simulink model "gm_CustArch_v13"  (R2020a)
settings: Solver=FixedStepDiscrete  StartTime=0.0  StopTime=840000  RelTol=1e-3
libraries: simulink x89, hdlsllib x54, hdlmdlgenlib x25
(part 2 of 3)

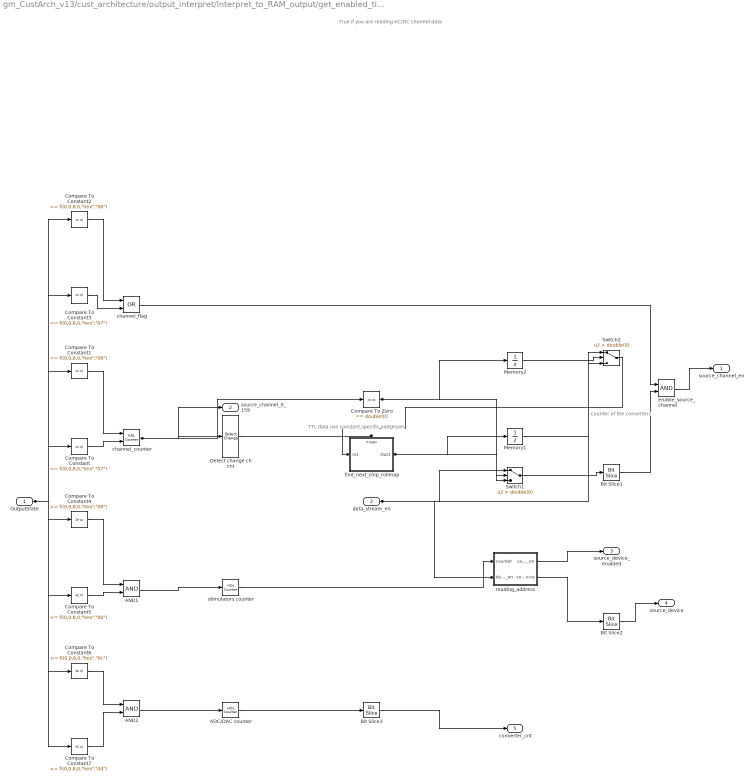
== system gm_CustArch_v13/cust_architecture/output_interpret/Interpret_to_RAM_output/get_enabled_timings  ==
  note: counter of the converters
  note: TTL data use constant specific addresses
  note: True if you are reading AC/DC channel data
  OutputState : Inport  OutDataTypeStr=uint8  PortDimensions=1  SampleTime=1
  data_stream_en : Inport  Port=2  OutDataTypeStr=uint8  PortDimensions=1  SampleTime=1
  ADC/DAC counter : hdlsllib/Sources/HDL Counter  CountType=Count limited  CountInit=double(0)  CountStep=double(1)  CountMax=double(7)  CountFromType=Initial value  CountFrom=double(0)  CountResetPort=off  CountLoadPort=off  CountEnbPort=on  CountDirPort=off  CountDataType=Unsigned  CountWordLen=8  CountFracLen=0  CountSampTime=1
  AND1 : Logic  AllPortsSameDT=off  OutDataTypeStr=boolean  SampleTime=1
  AND2 : Logic  AllPortsSameDT=off  OutDataTypeStr=boolean  SampleTime=1
  Bit Slice1 : hdlsllib/Logic and Bit Operations/Bit Slice  lidx=double(0)  ridx=double(0)
      settings: SourceProductBaseCode=SL
  Bit Slice2 : hdlsllib/Logic and Bit Operations/Bit Slice  lidx=double(2)  ridx=double(0)
      settings: SourceProductBaseCode=SL
  Bit Slice3 : hdlsllib/Logic and Bit Operations/Bit Slice  lidx=double(2)  ridx=double(0)
      settings: SourceProductBaseCode=SL
  Compare To Constant : simulink/Logic and Bit Operations/Compare To Constant  relop===  const="fi(0,0,8,0,\"hex\",\"07\")"  OutDataTypeStr=boolean
  Compare To Constant1 : simulink/Logic and Bit Operations/Compare To Constant  relop===  const="fi(0,0,8,0,\"hex\",\"08\")"  OutDataTypeStr=boolean
  Compare To Constant2 : simulink/Logic and Bit Operations/Compare To Constant  relop===  const="fi(0,0,8,0,\"hex\",\"06\")"  OutDataTypeStr=boolean
  Compare To Constant3 : simulink/Logic and Bit Operations/Compare To Constant  relop===  const="fi(0,0,8,0,\"hex\",\"07\")"  OutDataTypeStr=boolean
  Compare To Constant4 : simulink/Logic and Bit Operations/Compare To Constant  relop=>=  const="fi(0,0,8,0,\"hex\",\"08\")"  OutDataTypeStr=boolean
  Compare To Constant5 : simulink/Logic and Bit Operations/Compare To Constant  relop=<=  const="fi(0,0,8,0,\"hex\",\"0b\")"  OutDataTypeStr=boolean
  Compare To Constant6 : simulink/Logic and Bit Operations/Compare To Constant  relop=>=  const="fi(0,0,8,0,\"hex\",\"0c\")"  OutDataTypeStr=boolean
  Compare To Constant7 : simulink/Logic and Bit Operations/Compare To Constant  relop=<=  const="fi(0,0,8,0,\"hex\",\"0d\")"  OutDataTypeStr=boolean
  Compare To Zero : simulink/Logic and Bit Operations/Compare To Constant  relop===  const=double(0)  OutDataTypeStr=boolean
  Detect change ch cnt : simulink/Logic and Bit Operations/Detect Change  vinit=0  OutDataTypeStr=boolean
  Memory1 : UnitDelay  InitialCondition=double(0)  SampleTime=1
  Memory2 : UnitDelay  InitialCondition=double(0)  SampleTime=1
  Switch1 : Switch  Criteria=u2 > Threshold  Threshold=double(0)  OutDataTypeStr=uint8  SampleTime=1
  Switch2 : Switch  Criteria=u2 > Threshold  Threshold=double(0)  OutDataTypeStr=uint8  SampleTime=1
  channel_counter : hdlsllib/Sources/HDL Counter  CountType=Count limited  CountInit=double(0)  CountStep=double(1)  CountMax=double(159)  CountFromType=Initial value  CountFrom=double(0)  CountResetPort=on  CountLoadPort=off  CountEnbPort=on  CountDirPort=off  CountDataType=Unsigned  CountWordLen=8  CountFracLen=0  CountSampTime=1
  channel_flag : Logic  Operator=OR  AllPortsSameDT=off  OutDataTypeStr=boolean  SampleTime=1
  enable_source_channel : Logic  AllPortsSameDT=off  OutDataTypeStr=boolean  SampleTime=1
  find_next_chip_rollmap : Subsystem
  reading_address : Subsystem
  stimulators counter : hdlsllib/Sources/HDL Counter  CountType=Count limited  CountInit=double(0)  CountStep=double(1)  CountMax=double(7)  CountFromType=Initial value  CountFrom=double(0)  CountResetPort=off  CountLoadPort=off  CountEnbPort=on  CountDirPort=off  CountDataType=Unsigned  CountWordLen=8  CountFracLen=0  CountSampTime=1
  source_channel_en : Outport  VectorParamsAs1DForOutWhenUnconnected=off
  source_channel_0_159 : Outport  Port=2  OutMin=0  OutMax=159  OutDataTypeStr=uint8  VectorParamsAs1DForOutWhenUnconnected=off  LockScale=on
  source_device_enabled : Outport  Port=3  VectorParamsAs1DForOutWhenUnconnected=off
  source_device : Outport  Port=4  VectorParamsAs1DForOutWhenUnconnected=off
  converter_cnt : Outport  Port=5  VectorParamsAs1DForOutWhenUnconnected=off
  wires:
  OutputState/1 -> Compare To Constant7/1, Compare To Constant6/1, Compare To Constant5/1, Compare To Constant4/1, Compare To Constant3/1, Compare To Constant2/1, Compare To Constant1/1, Compare To Constant/1
  data_stream_en/1 -> Switch2/1, Switch1/1, reading_address/2(data_stream_en)
  ADC/DAC counter/1 -> Bit Slice3/1
  AND1/1 -> stimulators counter/1
  AND2/1 -> ADC/DAC counter/1
  Bit Slice1/1 -> enable_source_channel/2
  Bit Slice2/1 -> source_device/1
  Bit Slice3/1 -> converter_cnt/1
  Compare To Constant/1 -> channel_counter/2
  Compare To Constant1/1 -> channel_counter/1
  Compare To Constant2/1 -> channel_flag/1
  Compare To Constant3/1 -> channel_flag/2
  Compare To Constant4/1 -> AND1/1
  Compare To Constant5/1 -> AND1/2
  Compare To Constant6/1 -> AND2/1
  Compare To Constant7/1 -> AND2/2
  Compare To Zero/1 -> Switch1/2, Memory2/1
  Detect change ch cnt/1 -> find_next_chip_rollmap/Trigger
  Memory1/1 -> Switch2/3
  Memory2/1 -> Switch2/2
  Switch1/1 -> Bit Slice1/1
  Switch2/1 -> find_next_chip_rollmap/1(In1)
  channel_counter/1 -> Compare To Zero/1, Detect change ch cnt/1, source_channel_0_159/1
  channel_flag/1 -> enable_source_channel/1
  enable_source_channel/1 -> source_channel_en/1
  find_next_chip_rollmap/1(Out1) -> Switch1/3, Memory1/1
  reading_address/1(source_device_en) -> source_device_enabled/1
  reading_address/2(source_device) -> Bit Slice2/1
  stimulators counter/1 -> reading_address/1("counter ")

== system gm_CustArch_v13/cust_architecture/process_and_retrieve/Filter_ch1/digital_filter ==
  raw_input : Inport  OutDataTypeStr=uint16  PortDimensions=[8 1]  SampleTime=1  LockScale=on
  Enable : Inport  Port=2  OutDataTypeStr=boolean  SampleTime=1
  Add : Sum  Inputs=+-  AccumDataTypeStr=fixdt(1, 17, 0)  OutDataTypeStr=fixdt(1, 32, 16)  SampleTime=1
  Add1 : Sum  AccumDataTypeStr=fixdt(1, 38, 20)  OutDataTypeStr=uint16  SampleTime=1
  Add1_out1bypassMux : MultiPortSwitch  DataPortOrder=Zero-based contiguous  Inputs=2  zeroidx=on  OutDataTypeStr=uint16  SampleTime=1
  Constant : Constant  Value=32768  OutDataTypeStr=uint16  SampleTime=1
  Constant1 : Constant  Value=32768  OutDataTypeStr=uint16  SampleTime=1
  filter_output_bypass : UnitDelay  SampleTime=1
  highpass : Subsystem
  filter_output : Outport  InitialOutput=0  LockScale=on
  wires:
  Enable/1 -> Add1_out1bypassMux/1, highpass/2(Enable_out2)
  raw_input/1 -> Add/1
  Add/1 -> highpass/1(In)
  Add1/1 -> Add1_out1bypassMux/3
  Constant/1 -> Add/2
  Constant1/1 -> Add1/2
  highpass/1(Out) -> Add1/1
  Add1_out1bypassMux/1 -> filter_output_bypass/1, filter_output/1
  filter_output_bypass/1 -> Add1_out1bypassMux/2

== system gm_CustArch_v13/cust_architecture/input_interpret_store_retrieve/Interpret_to_RAM_input/interpret incoming data/condition to count DAC or ADC  ==
  fifo_write_to : Inport  OutDataTypeStr=boolean  PortDimensions=1  SampleTime=1
  input_state : Inport  Port=2  OutDataTypeStr=uint8  PortDimensions=1  SampleTime=1
  AND : Logic  AllPortsSameDT=off  OutDataTypeStr=boolean  SampleTime=1
  OR : Logic  Operator=OR  AllPortsSameDT=off  OutDataTypeStr=boolean  SampleTime=1
  is state_ADC : simulink/Logic and Bit Operations/Compare To Constant  relop===  const="fi(0,0,8,0,\"hex\",\"0d\")"  OutDataTypeStr=boolean
  is state_DAC : simulink/Logic and Bit Operations/Compare To Constant  relop===  const="fi(0,0,8,0,\"hex\",\"0c\")"  OutDataTypeStr=boolean
  Out1 : Outport  VectorParamsAs1DForOutWhenUnconnected=off
  wires:
  fifo_write_to/1 -> AND/1
  input_state/1 -> is state_DAC/1, is state_ADC/1
  AND/1 -> Out1/1
  OR/1 -> AND/2
  is state_ADC/1 -> OR/2
  is state_DAC/1 -> OR/1

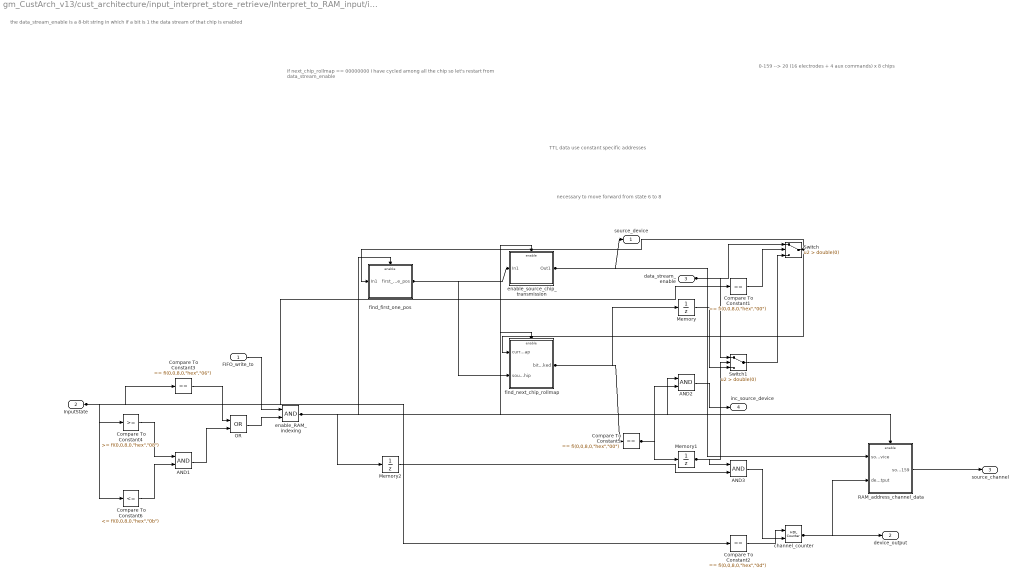
== system gm_CustArch_v13/cust_architecture/input_interpret_store_retrieve/Interpret_to_RAM_input/interpret incoming data/get_sources_and_RAM_addresses ==
  note: TTL data use constant specific addresses
  note: the data_stream_enable is a 8-bit string in which if a bit is 1 the data stream of that chip is enabled
  note: if next_chip_rollmap == 00000000 I have cycled among all the chip so let's restart from data_stream_enable
  note: 0-159 --> 20 (16 electrodes + 4 aux commands) x 8 chips
  note: necessary to move forward from state 6 to 8
  FIFO_write_to : Inport  OutDataTypeStr=boolean  PortDimensions=1  SampleTime=1
  InputState : Inport  Port=2  OutDataTypeStr=uint8  PortDimensions=1  SampleTime=1
  data_stream_enable : Inport  Port=3  OutDataTypeStr=uint8  PortDimensions=1  SampleTime=1
  AND1 : Logic  AllPortsSameDT=off  OutDataTypeStr=boolean  SampleTime=1
  AND2 : Logic  AllPortsSameDT=off  OutDataTypeStr=boolean  SampleTime=1
  AND3 : Logic  AllPortsSameDT=off  OutDataTypeStr=boolean  SampleTime=1
  Compare To Constant1 : simulink/Logic and Bit Operations/Compare To Constant  relop===  const="fi(0,0,8,0,\"hex\",\"00\")"  OutDataTypeStr=boolean
  Compare To Constant2 : simulink/Logic and Bit Operations/Compare To Constant  relop===  const="fi(0,0,8,0,\"hex\",\"0d\")"  OutDataTypeStr=boolean
  Compare To Constant3 : simulink/Logic and Bit Operations/Compare To Constant  relop===  const="fi(0,0,8,0,\"hex\",\"06\")"  OutDataTypeStr=boolean
  Compare To Constant4 : simulink/Logic and Bit Operations/Compare To Constant  relop=>=  const="fi(0,0,8,0,\"hex\",\"08\")"  OutDataTypeStr=boolean
  Compare To Constant5 : simulink/Logic and Bit Operations/Compare To Constant  relop===  const="fi(0,0,8,0,\"hex\",\"00\")"  OutDataTypeStr=boolean
  Compare To Constant6 : simulink/Logic and Bit Operations/Compare To Constant  relop=<=  const="fi(0,0,8,0,\"hex\",\"0b\")"  OutDataTypeStr=boolean
  Memory : UnitDelay  InitialCondition=double(0)  SampleTime=1
  Memory1 : UnitDelay  InitialCondition=double(0)  SampleTime=1
  Memory2 : UnitDelay  InitialCondition=double(0)  SampleTime=1
  OR : Logic  Operator=OR  AllPortsSameDT=off  OutDataTypeStr=boolean  SampleTime=1
  RAM_address_channel_data : Subsystem
  Switch : Switch  Criteria=u2 > Threshold  Threshold=double(0)  OutDataTypeStr=uint8  SampleTime=1
  Switch1 : Switch  Criteria=u2 > Threshold  Threshold=double(0)  OutDataTypeStr=uint8  SampleTime=1
  channel_counter : hdlsllib/Sources/HDL Counter  CountType=Count limited  CountInit=double(0)  CountStep=double(1)  CountMax=double(20)  CountFromType=Initial value  CountFrom=double(0)  CountResetPort=on  CountLoadPort=off  CountEnbPort=on  CountDirPort=off  CountDataType=Unsigned  CountWordLen=8  CountFracLen=0  CountSampTime=1
  enable_RAM_indexing : Logic  AllPortsSameDT=off  OutDataTypeStr=boolean  SampleTime=1
  enable_source_chip_transmission : Subsystem
  find_first_one_pos : Subsystem
  find_next_chip_rollmap : Subsystem
  source_device : Outport  VectorParamsAs1DForOutWhenUnconnected=off
  device_output : Outport  Port=2  VectorParamsAs1DForOutWhenUnconnected=off
  source_channel : Outport  Port=3  VectorParamsAs1DForOutWhenUnconnected=off
  inc_source_device : Outport  Port=4  VectorParamsAs1DForOutWhenUnconnected=off
  wires:
  FIFO_write_to/1 -> enable_RAM_indexing/1
  InputState/1 -> Compare To Constant6/1, Compare To Constant4/1, Compare To Constant3/1, Compare To Constant2/1, Compare To Constant1/1
  data_stream_enable/1 -> Switch1/1, Switch/1
  AND1/1 -> OR/2
  AND2/1 -> inc_source_device/1
  AND3/1 -> channel_counter/2
  Compare To Constant1/1 -> Switch/2
  Compare To Constant2/1 -> channel_counter/1
  Compare To Constant3/1 -> OR/1
  Compare To Constant4/1 -> AND1/1
  Compare To Constant5/1 -> AND2/2, Memory1/1
  Compare To Constant6/1 -> AND1/2
  Memory/1 -> Switch1/3
  Memory1/1 -> Switch1/2, AND3/1
  Memory2/1 -> AND3/2
  OR/1 -> enable_RAM_indexing/2
  RAM_address_channel_data/1(source_channel_0_159) -> source_channel/1
  Switch/1 -> find_next_chip_rollmap/1(curr_chip_rollmap), find_first_one_pos/1(In1)
  Switch1/1 -> Switch/3
  channel_counter/1 -> device_output/1, RAM_address_channel_data/2(dev_output)
  enable_RAM_indexing/1 -> AND2/1, Memory2/1, enable_source_chip_transmission/Enable, RAM_address_channel_data/Enable, find_next_chip_rollmap/Enable, find_first_one_pos/Enable
  enable_source_chip_transmission/1(Out1) -> source_device/1, RAM_address_channel_data/1(source_device)
  find_first_one_pos/1(first_one_pos) -> enable_source_chip_transmission/1(In1), find_next_chip_rollmap/2(source_chip)
  find_next_chip_rollmap/1(bit_masked) -> Compare To Constant5/1, Memory/1

== system gm_CustArch_v13/cust_architecture/output_interpret/Interpret_to_RAM_output/get_enabled_timings /find_next_chip_rollmap ==
  In1 : Inport  OutDataTypeStr=uint8  PortDimensions=1
  Trigger : TriggerPort  VariantControl=(inherit)  PortDimensions=1  OutDataTypeStr=boolean
  Bit Rotate : hdlsllib/Logic and Bit Operations/Bit Rotate  mode=Rotate Right  N=double(1)
      settings: SourceProductBaseCode=SL
  Out1 : Outport  InitialOutput=0  VectorParamsAs1DForOutWhenUnconnected=off
  wires:
  In1/1 -> Bit Rotate/1
  Bit Rotate/1 -> Out1/1

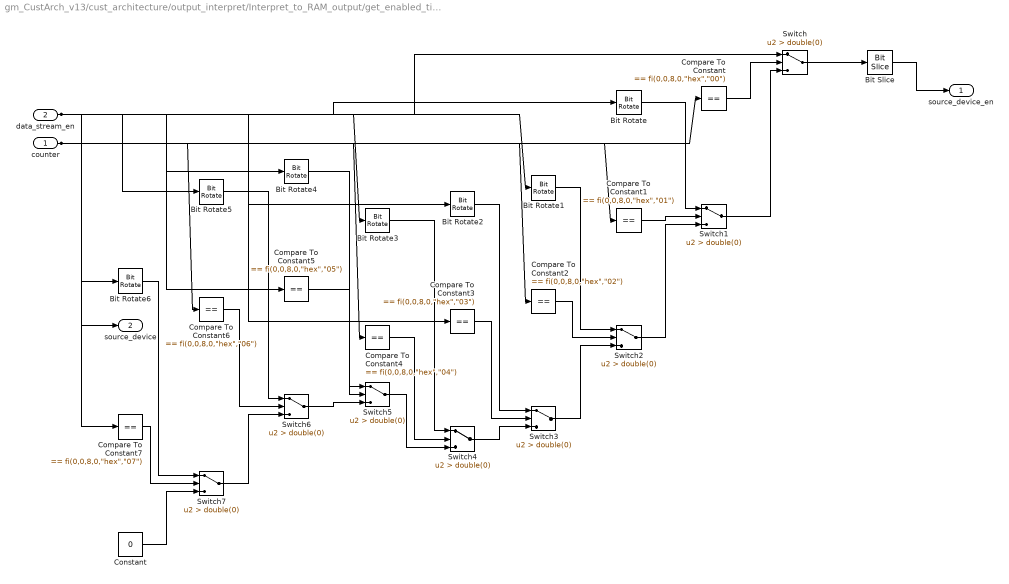
== system gm_CustArch_v13/cust_architecture/output_interpret/Interpret_to_RAM_output/get_enabled_timings /reading_address ==
  "counter " : Inport  OutDataTypeStr=uint8  PortDimensions=1  SampleTime=1
  data_stream_en : Inport  Port=2  OutDataTypeStr=uint8  PortDimensions=1  SampleTime=1
  Bit Rotate : hdlsllib/Logic and Bit Operations/Bit Rotate  mode=Rotate Right  N=double(1)
      settings: SourceProductBaseCode=SL
  Bit Rotate1 : hdlsllib/Logic and Bit Operations/Bit Rotate  mode=Rotate Right  N=double(2)
      settings: SourceProductBaseCode=SL
  Bit Rotate2 : hdlsllib/Logic and Bit Operations/Bit Rotate  mode=Rotate Right  N=double(3)
      settings: SourceProductBaseCode=SL
  Bit Rotate3 : hdlsllib/Logic and Bit Operations/Bit Rotate  mode=Rotate Right  N=double(4)
      settings: SourceProductBaseCode=SL
  Bit Rotate4 : hdlsllib/Logic and Bit Operations/Bit Rotate  mode=Rotate Right  N=double(5)
      settings: SourceProductBaseCode=SL
  Bit Rotate5 : hdlsllib/Logic and Bit Operations/Bit Rotate  mode=Rotate Right  N=double(6)
      settings: SourceProductBaseCode=SL
  Bit Rotate6 : hdlsllib/Logic and Bit Operations/Bit Rotate  mode=Rotate Right  N=double(7)
      settings: SourceProductBaseCode=SL
  Bit Slice : hdlsllib/Logic and Bit Operations/Bit Slice  lidx=double(0)  ridx=double(0)
      settings: SourceProductBaseCode=SL
  Compare To Constant : simulink/Logic and Bit Operations/Compare To Constant  relop===  const="fi(0,0,8,0,\"hex\",\"00\")"  OutDataTypeStr=boolean
  Compare To Constant1 : simulink/Logic and Bit Operations/Compare To Constant  relop===  const="fi(0,0,8,0,\"hex\",\"01\")"  OutDataTypeStr=boolean
  Compare To Constant2 : simulink/Logic and Bit Operations/Compare To Constant  relop===  const="fi(0,0,8,0,\"hex\",\"02\")"  OutDataTypeStr=boolean
  Compare To Constant3 : simulink/Logic and Bit Operations/Compare To Constant  relop===  const="fi(0,0,8,0,\"hex\",\"03\")"  OutDataTypeStr=boolean
  Compare To Constant4 : simulink/Logic and Bit Operations/Compare To Constant  relop===  const="fi(0,0,8,0,\"hex\",\"04\")"  OutDataTypeStr=boolean
  Compare To Constant5 : simulink/Logic and Bit Operations/Compare To Constant  relop===  const="fi(0,0,8,0,\"hex\",\"05\")"  OutDataTypeStr=boolean
  Compare To Constant6 : simulink/Logic and Bit Operations/Compare To Constant  relop===  const="fi(0,0,8,0,\"hex\",\"06\")"  OutDataTypeStr=boolean
  Compare To Constant7 : simulink/Logic and Bit Operations/Compare To Constant  relop===  const="fi(0,0,8,0,\"hex\",\"07\")"  OutDataTypeStr=boolean
  Constant : Constant  Value=0  OutDataTypeStr=uint8  SampleTime=1
  Switch{,1..7} (8 alike) : Switch  Criteria=u2 > Threshold  Threshold=double(0)  OutDataTypeStr=uint8  SampleTime=1
  source_device_en : Outport  VectorParamsAs1DForOutWhenUnconnected=off
  source_device : Outport  Port=2  VectorParamsAs1DForOutWhenUnconnected=off
  wires:
  "counter "/1 -> Compare To Constant7/1, Compare To Constant6/1, Compare To Constant5/1, Compare To Constant4/1, Compare To Constant3/1, Compare To Constant2/1, Compare To Constant1/1, Compare To Constant/1, source_device/1
  data_stream_en/1 -> Switch/1, Bit Rotate6/1, Bit Rotate5/1, Bit Rotate4/1, Bit Rotate3/1, Bit Rotate2/1, Bit Rotate1/1, Bit Rotate/1
  Bit Rotate/1 -> Switch1/1
  Bit Rotate1/1 -> Switch2/1
  Bit Rotate2/1 -> Switch3/1
  Bit Rotate3/1 -> Switch4/1
  Bit Rotate4/1 -> Switch5/1
  Bit Rotate5/1 -> Switch6/1
  Bit Rotate6/1 -> Switch7/1
  Bit Slice/1 -> source_device_en/1
  Compare To Constant/1 -> Switch/2
  Compare To Constant1/1 -> Switch1/2
  Compare To Constant2/1 -> Switch2/2
  Compare To Constant3/1 -> Switch3/2
  Compare To Constant4/1 -> Switch4/2
  Compare To Constant5/1 -> Switch5/2
  Compare To Constant6/1 -> Switch6/2
  Compare To Constant7/1 -> Switch7/2
  Constant/1 -> Switch7/3
  Switch/1 -> Bit Slice/1
  Switch1/1 -> Switch/3
  Switch2/1 -> Switch1/3
  Switch3/1 -> Switch2/3
  Switch4/1 -> Switch3/3
  Switch5/1 -> Switch4/3
  Switch6/1 -> Switch5/3
  Switch7/1 -> Switch6/3

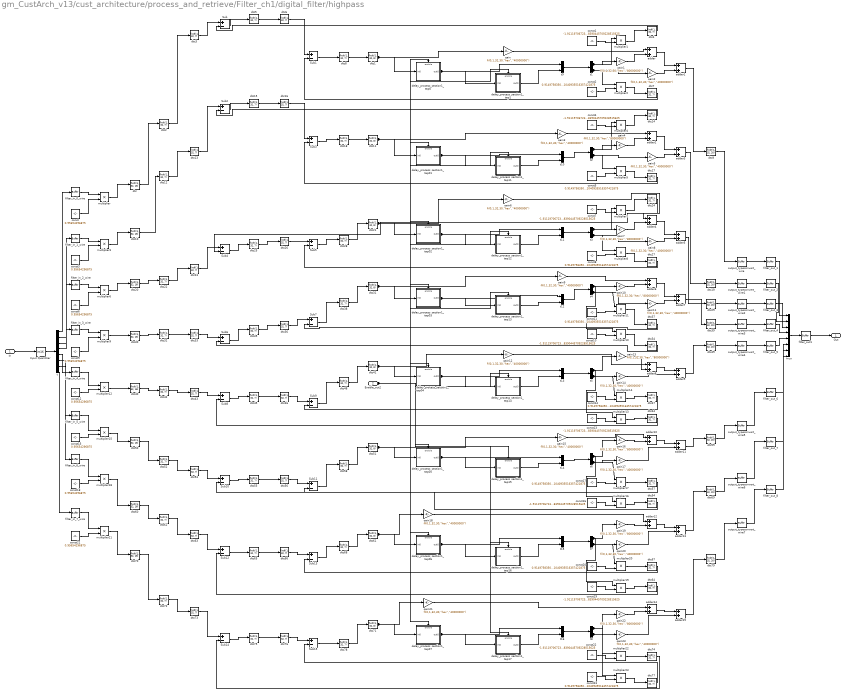
== system gm_CustArch_v13/cust_architecture/process_and_retrieve/Filter_ch1/digital_filter/highpass ==
  In : Inport  OutDataTypeStr=fixdt(1, 32, 16)  PortDimensions=[8 1]  SampleTime=1
  Enable_out2 : Inport  Port=2  OutDataTypeStr=boolean  SampleTime=1
  Input Quantizer : DataTypeConversion  OutDataTypeStr=int16  RndMeth=Round  SampleTime=1  SaturateOnIntegerOverflow=on
  Sub{,1..15} (16 alike) : Sum  Inputs=+-  OutDataTypeStr=fixdt(1, 33, 7)  RndMeth=Nearest  SaturateOnIntegerOverflow=on  SampleTime=1
  adder{,1..15} (16 alike) : Sum  OutDataTypeStr=fixdt(1, 32, 7)  RndMeth=Nearest  SaturateOnIntegerOverflow=on  SampleTime=1
  const{,3,6,9,12,15,18,21} (8 alike) : Constant  Value=0.95654296875  OutDataTypeStr=fixdt(1, 32, 15)  SampleTime=1
  const{1,4,7,10,13,16,19,22} (8 alike) : Constant  Value=-1.911197067238390445709228515625  OutDataTypeStr=fixdt(1, 32, 30)  SampleTime=1
  const{2,5,8,11,14,17,20,23} (8 alike) : Constant  Value=0.91497583501040935516357421875  OutDataTypeStr=fixdt(1, 32, 30)  SampleTime=1
  delay_process_section1_tap0 : Subsystem
      settings: MinAlgLoopOccurrences=on
  delay_process_section1_tap01 : Subsystem
      settings: MinAlgLoopOccurrences=on
  delay_process_section1_tap02 : Subsystem
      settings: MinAlgLoopOccurrences=on
  delay_process_section1_tap03 : Subsystem
      settings: MinAlgLoopOccurrences=on
  delay_process_section1_tap04 : Subsystem
      settings: MinAlgLoopOccurrences=on
  delay_process_section1_tap05 : Subsystem
      settings: MinAlgLoopOccurrences=on
  delay_process_section1_tap06 : Subsystem
      settings: MinAlgLoopOccurrences=on
  delay_process_section1_tap07 : Subsystem
      settings: MinAlgLoopOccurrences=on
  delay_process_section1_tap1 : Subsystem
      settings: MinAlgLoopOccurrences=on
  delay_process_section1_tap11 : Subsystem
      settings: MinAlgLoopOccurrences=on
  delay_process_section1_tap12 : Subsystem
      settings: MinAlgLoopOccurrences=on
  delay_process_section1_tap13 : Subsystem
      settings: MinAlgLoopOccurrences=on
  delay_process_section1_tap14 : Subsystem
      settings: MinAlgLoopOccurrences=on
  delay_process_section1_tap15 : Subsystem
      settings: MinAlgLoopOccurrences=on
  delay_process_section1_tap16 : Subsystem
      settings: MinAlgLoopOccurrences=on
  delay_process_section1_tap17 : Subsystem
      settings: MinAlgLoopOccurrences=on
  dtc{,10,20,30,40,50,60,70} (8 alike) : DataTypeConversion  OutDataTypeStr=fixdt(1, 32, 16)  RndMeth=Nearest  SampleTime=1  SaturateOnIntegerOverflow=on
  dtc{1,11,21,31,41,51,61,71} (8 alike) : DataTypeConversion  OutDataTypeStr=fixdt(1, 32, 8)  RndMeth=Nearest  SampleTime=1  SaturateOnIntegerOverflow=on
  dtc{2,12,22,32,42,52,62,72} (8 alike) : DataTypeConversion  OutDataTypeStr=fixdt(1, 32, 7)  RndMeth=Nearest  SampleTime=1  SaturateOnIntegerOverflow=on
  dtc{3..8,13..18,23..28,33..38,43..48,53..58,63..68,73..78} (48 alike) : DataTypeConversion  OutDataTypeStr=fixdt(1, 32, 7)  RndMeth=Nearest  SampleTime=1
  dtc{9,19,29,39,49,59,69,79} (8 alike) : DataTypeConversion  OutDataTypeStr=fixdt(1, 32, 20)  RndMeth=Nearest  SampleTime=1  SaturateOnIntegerOverflow=on
  filter_in_0_wire : hdlmdlgenlib/Buffer
      settings: SourceProductBaseCode=SL
  filter_in_1_wire : hdlmdlgenlib/Buffer
      settings: SourceProductBaseCode=SL
  filter_in_2_wire : hdlmdlgenlib/Buffer
      settings: SourceProductBaseCode=SL
  filter_in_3_wire : hdlmdlgenlib/Buffer
      settings: SourceProductBaseCode=SL
  filter_in_4_wire : hdlmdlgenlib/Buffer
      settings: SourceProductBaseCode=SL
  filter_in_5_wire : hdlmdlgenlib/Buffer
      settings: SourceProductBaseCode=SL
  filter_in_6_wire : hdlmdlgenlib/Buffer
      settings: SourceProductBaseCode=SL
  filter_in_7_wire : hdlmdlgenlib/Buffer
      settings: SourceProductBaseCode=SL
  filter_out1 : hdlmdlgenlib/Buffer
      settings: SourceProductBaseCode=SL
  filter_out_{1..8} (8 alike) : hdlmdlgenlib/Buffer
      settings: SourceProductBaseCode=SL
  gain{,2..3,5..6,8..9,11..12,14..15,17..18,20..21,23} (16 alike) : Gain  Gain="fi(0,1,32,30,\"hex\",\"40000000\")"  ParamDataTypeStr=fixdt(1, 32, 30)  OutDataTypeStr=fixdt(1, 32, 7)  RndMeth=Nearest  SampleTime=1
  gain{1,4,7,10,13,16,19,22} (8 alike) : Gain  Gain="fi(0,1,32,30,\"hex\",\"80000000\")"  ParamDataTypeStr=fixdt(1, 32, 30)  OutDataTypeStr=fixdt(1, 32, 7)  RndMeth=Nearest  SampleTime=1
  multiplier{,3,6,9,12,15,18,21} (8 alike) : Product  Inputs=**  OutDataTypeStr=fixdt(1, 64, 26)  RndMeth=Nearest  SampleTime=1
  multiplier{1..2,4..5,7..8,10..11,13..14,16..17,19..20,22..23} (16 alike) : Product  Inputs=**  OutDataTypeStr=fixdt(1, 32, 7)  RndMeth=Nearest  SampleTime=1
  mux : Mux  Inputs=8
  output_typeconvert_wire{,1..7} (8 alike) : hdlmdlgenlib/Buffer
      settings: SourceProductBaseCode=SL
  t : Demux  Outputs=8
  t{1..8} (8 alike) : Demux  Outputs=2
  t{9..16} (8 alike) : Mux  Inputs=2
  Out : Outport  InitialOutput=0
  wires:
  In/1 -> Input Quantizer/1
  Input Quantizer/1 -> t/1
  filter_out1/1 -> Out/1
  mux/1 -> filter_out1/1
  filter_in_0_wire/1 -> multiplier/1
  filter_out_1/1 -> mux/1
  filter_in_1_wire/1 -> multiplier3/1
  filter_out_2/1 -> mux/2
  filter_in_2_wire/1 -> multiplier6/1
  filter_out_3/1 -> mux/3
  filter_in_3_wire/1 -> multiplier9/1
  filter_out_4/1 -> mux/4
  filter_in_4_wire/1 -> multiplier12/1
  filter_out_5/1 -> mux/5
  filter_in_5_wire/1 -> multiplier15/1
  filter_out_6/1 -> mux/6
  filter_in_6_wire/1 -> multiplier18/1
  filter_out_7/1 -> mux/7
  filter_in_7_wire/1 -> multiplier21/1
  filter_out_8/1 -> mux/8
  t/1 -> filter_in_0_wire/1
  t/2 -> filter_in_1_wire/1
  t/3 -> filter_in_2_wire/1
  t/4 -> filter_in_3_wire/1
  t/5 -> filter_in_4_wire/1
  t/6 -> filter_in_5_wire/1
  t/7 -> filter_in_6_wire/1
  t/8 -> filter_in_7_wire/1
  output_typeconvert_wire/1 -> filter_out_1/1
  const/1 -> multiplier/2
  multiplier/1 -> dtc/1
  const1/1 -> multiplier1/2
  const2/1 -> multiplier2/2
  dtc/1 -> dtc2/1
  dtc8/1 -> dtc1/1
  dtc5/1 -> dtc6/1
  adder1/1 -> dtc9/1
  adder/1 -> adder1/1
  dtc1/1 -> delay_process_section1_tap0/1(in0), gain/1
  t9/1 -> t1/1
  t1/1 -> multiplier1/1, gain1/1
  t1/2 -> multiplier2/1, gain2/1
  dtc2/1 -> dtc3/1
  multiplier1/1 -> dtc4/1
  multiplier2/1 -> dtc7/1
  gain/1 -> adder/1
  gain1/1 -> adder/2
  gain2/1 -> adder1/2
  dtc3/1 -> Sub/1
  dtc4/1 -> Sub/2
  Sub/1 -> dtc5/1
  dtc6/1 -> Sub1/1
  dtc7/1 -> Sub1/2
  Sub1/1 -> dtc8/1
  dtc9/1 -> output_typeconvert_wire/1
  output_typeconvert_wire1/1 -> filter_out_2/1
  const3/1 -> multiplier3/2
  multiplier3/1 -> dtc10/1
  const4/1 -> multiplier4/2
  const5/1 -> multiplier5/2
  dtc10/1 -> dtc12/1
  dtc18/1 -> dtc11/1
  dtc15/1 -> dtc16/1
  adder3/1 -> dtc19/1
  adder2/1 -> adder3/1
  dtc11/1 -> delay_process_section1_tap01/1(in0), gain3/1
  t10/1 -> t2/1
  t2/1 -> multiplier4/1, gain4/1
  t2/2 -> multiplier5/1, gain5/1
  dtc12/1 -> dtc13/1
  multiplier4/1 -> dtc14/1
  multiplier5/1 -> dtc17/1
  gain3/1 -> adder2/1
  gain4/1 -> adder2/2
  gain5/1 -> adder3/2
  dtc13/1 -> Sub2/1
  dtc14/1 -> Sub2/2
  Sub2/1 -> dtc15/1
  dtc16/1 -> Sub3/1
  dtc17/1 -> Sub3/2
  Sub3/1 -> dtc18/1
  dtc19/1 -> output_typeconvert_wire1/1
  output_typeconvert_wire2/1 -> filter_out_3/1
  const6/1 -> multiplier6/2
  multiplier6/1 -> dtc20/1
  const7/1 -> multiplier7/2
  const8/1 -> multiplier8/2
  dtc20/1 -> dtc22/1
  dtc28/1 -> dtc21/1
  dtc25/1 -> dtc26/1
  adder5/1 -> dtc29/1
  adder4/1 -> adder5/1
  dtc21/1 -> delay_process_section1_tap02/1(in0), gain6/1
  t11/1 -> t3/1
  t3/1 -> multiplier7/1, gain7/1
  t3/2 -> multiplier8/1, gain8/1
  dtc22/1 -> dtc23/1
  multiplier7/1 -> dtc24/1
  multiplier8/1 -> dtc27/1
  gain6/1 -> adder4/1
  gain7/1 -> adder4/2
  gain8/1 -> adder5/2
  dtc23/1 -> Sub4/1
  dtc24/1 -> Sub4/2
  Sub4/1 -> dtc25/1
  dtc26/1 -> Sub5/1
  dtc27/1 -> Sub5/2
  Sub5/1 -> dtc28/1
  dtc29/1 -> output_typeconvert_wire2/1
  output_typeconvert_wire3/1 -> filter_out_4/1
  const9/1 -> multiplier9/2
  multiplier9/1 -> dtc30/1
  const10/1 -> multiplier10/2
  const11/1 -> multiplier11/2
  dtc30/1 -> dtc32/1
  dtc38/1 -> dtc31/1
  dtc35/1 -> dtc36/1
  adder7/1 -> dtc39/1
  adder6/1 -> adder7/1
  dtc31/1 -> delay_process_section1_tap03/1(in0), gain9/1
  t12/1 -> t4/1
  t4/1 -> multiplier10/1, gain10/1
  t4/2 -> multiplier11/1, gain11/1
  dtc32/1 -> dtc33/1
  multiplier10/1 -> dtc34/1
  multiplier11/1 -> dtc37/1
  gain9/1 -> adder6/1
  gain10/1 -> adder6/2
  gain11/1 -> adder7/2
  dtc33/1 -> Sub6/1
  dtc34/1 -> Sub6/2
  Sub6/1 -> dtc35/1
  dtc36/1 -> Sub7/1
  dtc37/1 -> Sub7/2
  Sub7/1 -> dtc38/1
  dtc39/1 -> output_typeconvert_wire3/1
  output_typeconvert_wire4/1 -> filter_out_5/1
  const12/1 -> multiplier12/2
  multiplier12/1 -> dtc40/1
  const13/1 -> multiplier13/2
  const14/1 -> multiplier14/2
  dtc40/1 -> dtc42/1
  dtc48/1 -> dtc41/1
  dtc45/1 -> dtc46/1
  adder9/1 -> dtc49/1
  adder8/1 -> adder9/1
  dtc41/1 -> delay_process_section1_tap04/1(in0), gain12/1
  t13/1 -> t5/1
  t5/1 -> multiplier13/1, gain13/1
  t5/2 -> multiplier14/1, gain14/1
  dtc42/1 -> dtc43/1
  multiplier13/1 -> dtc44/1
  multiplier14/1 -> dtc47/1
  gain12/1 -> adder8/1
  gain13/1 -> adder8/2
  gain14/1 -> adder9/2
  dtc43/1 -> Sub8/1
  dtc44/1 -> Sub8/2
  Sub8/1 -> dtc45/1
  dtc46/1 -> Sub9/1
  dtc47/1 -> Sub9/2
  Sub9/1 -> dtc48/1
  dtc49/1 -> output_typeconvert_wire4/1
  output_typeconvert_wire5/1 -> filter_out_6/1
  const15/1 -> multiplier15/2
  multiplier15/1 -> dtc50/1
  const16/1 -> multiplier16/2
  const17/1 -> multiplier17/2
  dtc50/1 -> dtc52/1
  dtc58/1 -> dtc51/1
  dtc55/1 -> dtc56/1
  adder11/1 -> dtc59/1
  adder10/1 -> adder11/1
  dtc51/1 -> delay_process_section1_tap05/1(in0), gain15/1
  t14/1 -> t6/1
  t6/1 -> multiplier16/1, gain16/1
  t6/2 -> multiplier17/1, gain17/1
  dtc52/1 -> dtc53/1
  multiplier16/1 -> dtc54/1
  multiplier17/1 -> dtc57/1
  gain15/1 -> adder10/1
  gain16/1 -> adder10/2
  gain17/1 -> adder11/2
  dtc53/1 -> Sub10/1
  dtc54/1 -> Sub10/2
  Sub10/1 -> dtc55/1
  dtc56/1 -> Sub11/1
  dtc57/1 -> Sub11/2
  Sub11/1 -> dtc58/1
  dtc59/1 -> output_typeconvert_wire5/1
  output_typeconvert_wire6/1 -> filter_out_7/1
  const18/1 -> multiplier18/2
  multiplier18/1 -> dtc60/1
  const19/1 -> multiplier19/2
  const20/1 -> multiplier20/2
  dtc60/1 -> dtc62/1
  dtc68/1 -> dtc61/1
  dtc65/1 -> dtc66/1
  adder13/1 -> dtc69/1
  adder12/1 -> adder13/1
  dtc61/1 -> delay_process_section1_tap06/1(in0), gain18/1
  t15/1 -> t7/1
  t7/1 -> multiplier19/1, gain19/1
  t7/2 -> multiplier20/1, gain20/1
  dtc62/1 -> dtc63/1
  multiplier19/1 -> dtc64/1
  multiplier20/1 -> dtc67/1
  gain18/1 -> adder12/1
  gain19/1 -> adder12/2
  gain20/1 -> adder13/2
  dtc63/1 -> Sub12/1
  dtc64/1 -> Sub12/2
  Sub12/1 -> dtc65/1
  dtc66/1 -> Sub13/1
  dtc67/1 -> Sub13/2
  Sub13/1 -> dtc68/1
  dtc69/1 -> output_typeconvert_wire6/1
  output_typeconvert_wire7/1 -> filter_out_8/1
  const21/1 -> multiplier21/2
  multiplier21/1 -> dtc70/1
  const22/1 -> multiplier22/2
  const23/1 -> multiplier23/2
  dtc70/1 -> dtc72/1
  dtc78/1 -> dtc71/1
  dtc75/1 -> dtc76/1
  adder15/1 -> dtc79/1
  adder14/1 -> adder15/1
  dtc71/1 -> delay_process_section1_tap07/1(in0), gain21/1
  t16/1 -> t8/1
  t8/1 -> gain22/1, multiplier22/1
  t8/2 -> gain23/1, multiplier23/1
  dtc72/1 -> dtc73/1
  multiplier22/1 -> dtc74/1
  multiplier23/1 -> dtc77/1
  gain21/1 -> adder14/1
  gain22/1 -> adder14/2
  gain23/1 -> adder15/2
  dtc73/1 -> Sub14/1
  dtc74/1 -> Sub14/2
  Sub14/1 -> dtc75/1
  dtc76/1 -> Sub15/1
  dtc77/1 -> Sub15/2
  Sub15/1 -> dtc78/1
  dtc79/1 -> output_typeconvert_wire7/1
  delay_process_section1_tap0/1(out0) -> delay_process_section1_tap1/1(in0), t9/1
  delay_process_section1_tap1/1(out0) -> t9/2
  delay_process_section1_tap01/1(out0) -> delay_process_section1_tap11/1(in0), t10/1
  delay_process_section1_tap11/1(out0) -> t10/2
  delay_process_section1_tap02/1(out0) -> delay_process_section1_tap12/1(in0), t11/1
  delay_process_section1_tap12/1(out0) -> t11/2
  delay_process_section1_tap03/1(out0) -> delay_process_section1_tap13/1(in0), t12/1
  delay_process_section1_tap13/1(out0) -> t12/2
  delay_process_section1_tap04/1(out0) -> delay_process_section1_tap14/1(in0), t13/1
  delay_process_section1_tap14/1(out0) -> t13/2
  delay_process_section1_tap05/1(out0) -> delay_process_section1_tap15/1(in0), t14/1
  delay_process_section1_tap15/1(out0) -> t14/2
  delay_process_section1_tap06/1(out0) -> delay_process_section1_tap16/1(in0), t15/1
  delay_process_section1_tap16/1(out0) -> t15/2
  delay_process_section1_tap07/1(out0) -> delay_process_section1_tap17/1(in0), t16/1
  delay_process_section1_tap17/1(out0) -> t16/2
  Enable_out2/1 -> delay_process_section1_tap17/Enable, delay_process_section1_tap07/Enable, delay_process_section1_tap16/Enable, delay_process_section1_tap06/Enable, delay_process_section1_tap15/Enable, delay_process_section1_tap05/Enable, delay_process_section1_tap14/Enable, delay_process_section1_tap04/Enable, delay_process_section1_tap13/Enable, delay_process_section1_tap03/Enable, delay_process_section1_tap12/Enable, delay_process_section1_tap02/Enable, delay_process_section1_tap11/Enable, delay_process_section1_tap01/Enable, delay_process_section1_tap1/Enable, delay_process_section1_tap0/Enable

== system gm_CustArch_v13/cust_architecture/input_interpret_store_retrieve/Interpret_to_RAM_input/interpret incoming data/get_sources_and_RAM_addresses/RAM_address_channel_data ==
  source_device : Inport  OutDataTypeStr=uint8  PortDimensions=1  SampleTime=1
  dev_output : Inport  Port=2  OutDataTypeStr=uint8  PortDimensions=1  SampleTime=1
  Enable : EnablePort  OutDataTypeStr=boolean
  Bit Concat : hdlsllib/Logic and Bit Operations/Bit Concat  numInputs=2
  Bit Slice : hdlsllib/Logic and Bit Operations/Bit Slice  lidx=double(4)  ridx=double(0)
      settings: SourceProductBaseCode=SL
  Bit Slice1 : hdlsllib/Logic and Bit Operations/Bit Slice  lidx=double(2)  ridx=double(0)
      settings: SourceProductBaseCode=SL
  source_channel_0_159 : Outport  InitialOutput=0  VectorParamsAs1DForOutWhenUnconnected=off
  wires:
  source_device/1 -> Bit Slice1/1
  dev_output/1 -> Bit Slice/1
  Bit Concat/1 -> source_channel_0_159/1
  Bit Slice/1 -> Bit Concat/1
  Bit Slice1/1 -> Bit Concat/2

== system gm_CustArch_v13/cust_architecture/input_interpret_store_retrieve/Interpret_to_RAM_input/interpret incoming data/get_sources_and_RAM_addresses/enable_source_chip_transmission ==
  In1 : Inport  OutDataTypeStr=uint8  PortDimensions=1  SampleTime=1
  Enable : EnablePort  OutDataTypeStr=boolean
  Out1 : Outport  InitialOutput=0  VectorParamsAs1DForOutWhenUnconnected=off
  wires:
  In1/1 -> Out1/1

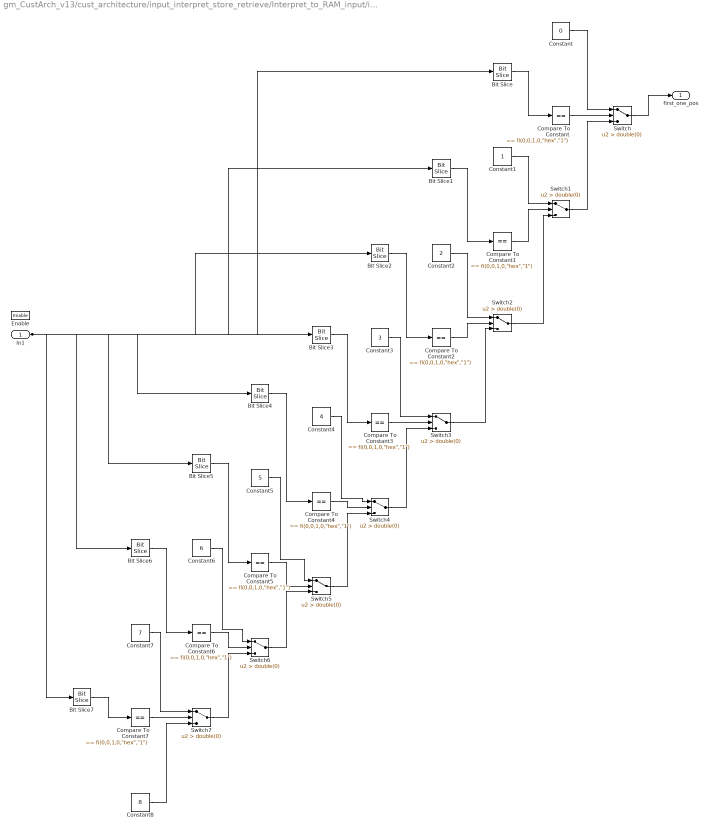
== system gm_CustArch_v13/cust_architecture/input_interpret_store_retrieve/Interpret_to_RAM_input/interpret incoming data/get_sources_and_RAM_addresses/find_first_one_pos ==
  In1 : Inport  OutDataTypeStr=uint8  PortDimensions=1  SampleTime=1
  Enable : EnablePort  OutDataTypeStr=boolean
  Bit Slice : hdlsllib/Logic and Bit Operations/Bit Slice  lidx=double(0)  ridx=double(0)
      settings: SourceProductBaseCode=SL
  Bit Slice1 : hdlsllib/Logic and Bit Operations/Bit Slice  lidx=double(1)  ridx=double(1)
      settings: SourceProductBaseCode=SL
  Bit Slice2 : hdlsllib/Logic and Bit Operations/Bit Slice  lidx=double(2)  ridx=double(2)
      settings: SourceProductBaseCode=SL
  Bit Slice3 : hdlsllib/Logic and Bit Operations/Bit Slice  lidx=double(3)  ridx=double(3)
      settings: SourceProductBaseCode=SL
  Bit Slice4 : hdlsllib/Logic and Bit Operations/Bit Slice  lidx=double(4)  ridx=double(4)
      settings: SourceProductBaseCode=SL
  Bit Slice5 : hdlsllib/Logic and Bit Operations/Bit Slice  lidx=double(5)  ridx=double(5)
      settings: SourceProductBaseCode=SL
  Bit Slice6 : hdlsllib/Logic and Bit Operations/Bit Slice  lidx=double(6)  ridx=double(6)
      settings: SourceProductBaseCode=SL
  Bit Slice7 : hdlsllib/Logic and Bit Operations/Bit Slice  lidx=double(7)  ridx=double(7)
      settings: SourceProductBaseCode=SL
  Compare To Constant{,1..7} (8 alike) : simulink/Logic and Bit Operations/Compare To Constant  relop===  const="fi(0,0,1,0,\"hex\",\"1\")"  OutDataTypeStr=boolean
  Constant : Constant  Value=0  OutDataTypeStr=uint8  SampleTime=1
  Constant1 : Constant  OutDataTypeStr=uint8  SampleTime=1
  Constant2 : Constant  Value=2  OutDataTypeStr=uint8  SampleTime=1
  Constant3 : Constant  Value=3  OutDataTypeStr=uint8  SampleTime=1
  Constant4 : Constant  Value=4  OutDataTypeStr=uint8  SampleTime=1
  Constant5 : Constant  Value=5  OutDataTypeStr=uint8  SampleTime=1
  Constant6 : Constant  Value=6  OutDataTypeStr=uint8  SampleTime=1
  Constant7 : Constant  Value=7  OutDataTypeStr=uint8  SampleTime=1
  Constant8 : Constant  Value=8  OutDataTypeStr=uint8  SampleTime=1
  Switch{,1..7} (8 alike) : Switch  Criteria=u2 > Threshold  Threshold=double(0)  OutDataTypeStr=uint8  SampleTime=1
  first_one_pos : Outport  InitialOutput=0  VectorParamsAs1DForOutWhenUnconnected=off
  wires:
  In1/1 -> Bit Slice7/1, Bit Slice6/1, Bit Slice5/1, Bit Slice4/1, Bit Slice3/1, Bit Slice2/1, Bit Slice1/1, Bit Slice/1
  Bit Slice/1 -> Compare To Constant/1
  Bit Slice1/1 -> Compare To Constant1/1
  Bit Slice2/1 -> Compare To Constant2/1
  Bit Slice3/1 -> Compare To Constant3/1
  Bit Slice4/1 -> Compare To Constant4/1
  Bit Slice5/1 -> Compare To Constant5/1
  Bit Slice6/1 -> Compare To Constant6/1
  Bit Slice7/1 -> Compare To Constant7/1
  Compare To Constant/1 -> Switch/2
  Compare To Constant1/1 -> Switch1/2
  Compare To Constant2/1 -> Switch2/2
  Compare To Constant3/1 -> Switch3/2
  Compare To Constant4/1 -> Switch4/2
  Compare To Constant5/1 -> Switch5/2
  Compare To Constant6/1 -> Switch6/2
  Compare To Constant7/1 -> Switch7/2
  Constant/1 -> Switch/1
  Constant1/1 -> Switch1/1
  Constant2/1 -> Switch2/1
  Constant3/1 -> Switch3/1
  Constant4/1 -> Switch4/1
  Constant5/1 -> Switch5/1
  Constant6/1 -> Switch6/1
  Constant7/1 -> Switch7/1
  Constant8/1 -> Switch7/3
  Switch/1 -> first_one_pos/1
  Switch1/1 -> Switch/3
  Switch2/1 -> Switch1/3
  Switch3/1 -> Switch2/3
  Switch4/1 -> Switch3/3
  Switch5/1 -> Switch4/3
  Switch6/1 -> Switch5/3
  Switch7/1 -> Switch6/3

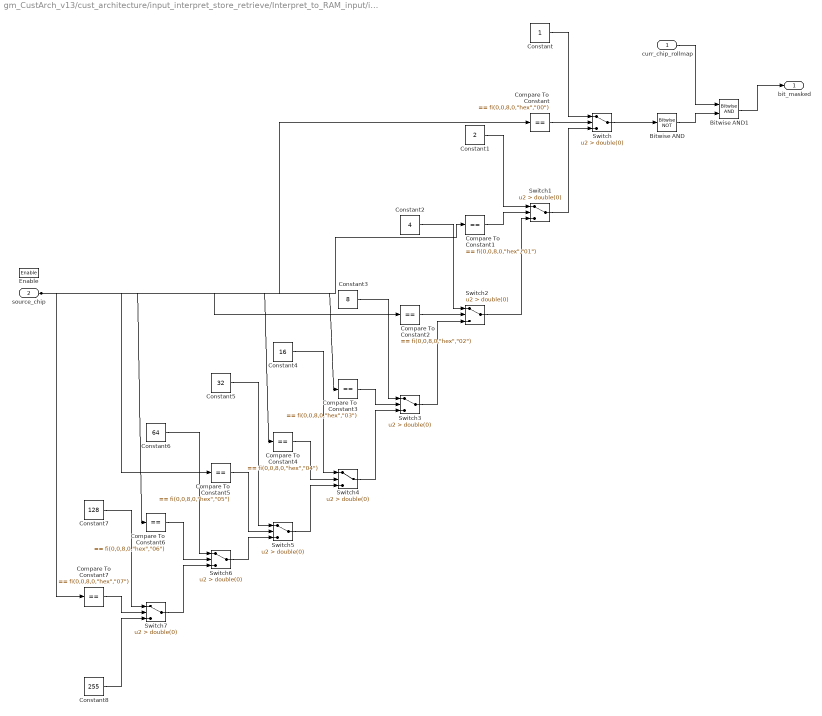
== system gm_CustArch_v13/cust_architecture/input_interpret_store_retrieve/Interpret_to_RAM_input/interpret incoming data/get_sources_and_RAM_addresses/find_next_chip_rollmap ==
  curr_chip_rollmap : Inport  OutDataTypeStr=uint8  PortDimensions=1  SampleTime=1
  source_chip : Inport  Port=2  OutDataTypeStr=uint8  PortDimensions=1  SampleTime=1
  Enable : EnablePort  OutDataTypeStr=boolean
  Bitwise AND : simulink/Logic and Bit Operations/Bitwise Operator  logicop=NOT  UseBitMask=off  BitMask=double(0)  BitMaskRealWorld=Real World Value
  Bitwise AND1 : simulink/Logic and Bit Operations/Bitwise Operator  logicop=AND  UseBitMask=off  NumInputPorts=2  BitMask=double(0)  BitMaskRealWorld=Real World Value
  Compare To Constant : simulink/Logic and Bit Operations/Compare To Constant  relop===  const="fi(0,0,8,0,\"hex\",\"00\")"  OutDataTypeStr=boolean
  Compare To Constant1 : simulink/Logic and Bit Operations/Compare To Constant  relop===  const="fi(0,0,8,0,\"hex\",\"01\")"  OutDataTypeStr=boolean
  Compare To Constant2 : simulink/Logic and Bit Operations/Compare To Constant  relop===  const="fi(0,0,8,0,\"hex\",\"02\")"  OutDataTypeStr=boolean
  Compare To Constant3 : simulink/Logic and Bit Operations/Compare To Constant  relop===  const="fi(0,0,8,0,\"hex\",\"03\")"  OutDataTypeStr=boolean
  Compare To Constant4 : simulink/Logic and Bit Operations/Compare To Constant  relop===  const="fi(0,0,8,0,\"hex\",\"04\")"  OutDataTypeStr=boolean
  Compare To Constant5 : simulink/Logic and Bit Operations/Compare To Constant  relop===  const="fi(0,0,8,0,\"hex\",\"05\")"  OutDataTypeStr=boolean
  Compare To Constant6 : simulink/Logic and Bit Operations/Compare To Constant  relop===  const="fi(0,0,8,0,\"hex\",\"06\")"  OutDataTypeStr=boolean
  Compare To Constant7 : simulink/Logic and Bit Operations/Compare To Constant  relop===  const="fi(0,0,8,0,\"hex\",\"07\")"  OutDataTypeStr=boolean
  Constant : Constant  OutDataTypeStr=uint8  SampleTime=1
  Constant1 : Constant  Value=2  OutDataTypeStr=uint8  SampleTime=1
  Constant2 : Constant  Value=4  OutDataTypeStr=uint8  SampleTime=1
  Constant3 : Constant  Value=8  OutDataTypeStr=uint8  SampleTime=1
  Constant4 : Constant  Value=16  OutDataTypeStr=uint8  SampleTime=1
  Constant5 : Constant  Value=32  OutDataTypeStr=uint8  SampleTime=1
  Constant6 : Constant  Value=64  OutDataTypeStr=uint8  SampleTime=1
  Constant7 : Constant  Value=128  OutDataTypeStr=uint8  SampleTime=1
  Constant8 : Constant  Value=255  OutDataTypeStr=uint8  SampleTime=1
  Switch{,1..7} (8 alike) : Switch  Criteria=u2 > Threshold  Threshold=double(0)  OutDataTypeStr=uint8  SampleTime=1
  bit_masked : Outport  InitialOutput=0  VectorParamsAs1DForOutWhenUnconnected=off
  wires:
  curr_chip_rollmap/1 -> Bitwise AND1/1
  source_chip/1 -> Compare To Constant7/1, Compare To Constant6/1, Compare To Constant5/1, Compare To Constant4/1, Compare To Constant3/1, Compare To Constant2/1, Compare To Constant1/1, Compare To Constant/1
  Bitwise AND/1 -> Bitwise AND1/2
  Bitwise AND1/1 -> bit_masked/1
  Compare To Constant/1 -> Switch/2
  Compare To Constant1/1 -> Switch1/2
  Compare To Constant2/1 -> Switch2/2
  Compare To Constant3/1 -> Switch3/2
  Compare To Constant4/1 -> Switch4/2
  Compare To Constant5/1 -> Switch5/2
  Compare To Constant6/1 -> Switch6/2
  Compare To Constant7/1 -> Switch7/2
  Constant/1 -> Switch/1
  Constant1/1 -> Switch1/1
  Constant2/1 -> Switch2/1
  Constant3/1 -> Switch3/1
  Constant4/1 -> Switch4/1
  Constant5/1 -> Switch5/1
  Constant6/1 -> Switch6/1
  Constant7/1 -> Switch7/1
  Constant8/1 -> Switch7/3
  Switch/1 -> Bitwise AND/1
  Switch1/1 -> Switch/3
  Switch2/1 -> Switch1/3
  Switch3/1 -> Switch2/3
  Switch4/1 -> Switch3/3
  Switch5/1 -> Switch4/3
  Switch6/1 -> Switch5/3
  Switch7/1 -> Switch6/3

== system gm_CustArch_v13/cust_architecture/process_and_retrieve/Filter_ch1/digital_filter/highpass/delay_process_section1_tap0 ==
  in0 : Inport  OutDataTypeStr=fixdt(1, 32, 8)  SampleTime=1
  Enable_out2 : EnablePort  OutDataTypeStr=boolean
  delay_process_section1_tap0 : Delay  DelayLength=double(1)
  out0 : Outport  OutDataTypeStr=fixdt(1, 32, 8)  InitialOutput=0
  wires:
  delay_process_section1_tap0/1 -> out0/1
  in0/1 -> delay_process_section1_tap0/1

== system gm_CustArch_v13/cust_architecture/process_and_retrieve/Filter_ch1/digital_filter/highpass/delay_process_section1_tap01 ==
  in0 : Inport  OutDataTypeStr=fixdt(1, 32, 8)  SampleTime=1
  Enable_out2 : EnablePort  OutDataTypeStr=boolean
  delay_process_section1_tap0 : Delay  DelayLength=double(1)
  out0 : Outport  OutDataTypeStr=fixdt(1, 32, 8)  InitialOutput=0
  wires:
  delay_process_section1_tap0/1 -> out0/1
  in0/1 -> delay_process_section1_tap0/1

== system gm_CustArch_v13/cust_architecture/process_and_retrieve/Filter_ch1/digital_filter/highpass/delay_process_section1_tap02 ==
  in0 : Inport  OutDataTypeStr=fixdt(1, 32, 8)  SampleTime=1
  Enable_out2 : EnablePort  OutDataTypeStr=boolean
  delay_process_section1_tap0 : Delay  DelayLength=double(1)
  out0 : Outport  OutDataTypeStr=fixdt(1, 32, 8)  InitialOutput=0
  wires:
  delay_process_section1_tap0/1 -> out0/1
  in0/1 -> delay_process_section1_tap0/1

== system gm_CustArch_v13/cust_architecture/process_and_retrieve/Filter_ch1/digital_filter/highpass/delay_process_section1_tap03 ==
  in0 : Inport  OutDataTypeStr=fixdt(1, 32, 8)  SampleTime=1
  Enable_out2 : EnablePort  OutDataTypeStr=boolean
  delay_process_section1_tap0 : Delay  DelayLength=double(1)
  out0 : Outport  OutDataTypeStr=fixdt(1, 32, 8)  InitialOutput=0
  wires:
  delay_process_section1_tap0/1 -> out0/1
  in0/1 -> delay_process_section1_tap0/1

== system gm_CustArch_v13/cust_architecture/process_and_retrieve/Filter_ch1/digital_filter/highpass/delay_process_section1_tap04 ==
  in0 : Inport  OutDataTypeStr=fixdt(1, 32, 8)  SampleTime=1
  Enable_out2 : EnablePort  OutDataTypeStr=boolean
  delay_process_section1_tap0 : Delay  DelayLength=double(1)
  out0 : Outport  OutDataTypeStr=fixdt(1, 32, 8)  InitialOutput=0
  wires:
  delay_process_section1_tap0/1 -> out0/1
  in0/1 -> delay_process_section1_tap0/1

== system gm_CustArch_v13/cust_architecture/process_and_retrieve/Filter_ch1/digital_filter/highpass/delay_process_section1_tap05 ==
  in0 : Inport  OutDataTypeStr=fixdt(1, 32, 8)  SampleTime=1
  Enable_out2 : EnablePort  OutDataTypeStr=boolean
  delay_process_section1_tap0 : Delay  DelayLength=double(1)
  out0 : Outport  OutDataTypeStr=fixdt(1, 32, 8)  InitialOutput=0
  wires:
  delay_process_section1_tap0/1 -> out0/1
  in0/1 -> delay_process_section1_tap0/1

== system gm_CustArch_v13/cust_architecture/process_and_retrieve/Filter_ch1/digital_filter/highpass/delay_process_section1_tap06 ==
  in0 : Inport  OutDataTypeStr=fixdt(1, 32, 8)  SampleTime=1
  Enable_out2 : EnablePort  OutDataTypeStr=boolean
  delay_process_section1_tap0 : Delay  DelayLength=double(1)
  out0 : Outport  OutDataTypeStr=fixdt(1, 32, 8)  InitialOutput=0
  wires:
  delay_process_section1_tap0/1 -> out0/1
  in0/1 -> delay_process_section1_tap0/1

== system gm_CustArch_v13/cust_architecture/process_and_retrieve/Filter_ch1/digital_filter/highpass/delay_process_section1_tap07 ==
  in0 : Inport  OutDataTypeStr=fixdt(1, 32, 8)  SampleTime=1
  Enable_out2 : EnablePort  OutDataTypeStr=boolean
  delay_process_section1_tap0 : Delay  DelayLength=double(1)
  out0 : Outport  OutDataTypeStr=fixdt(1, 32, 8)  InitialOutput=0
  wires:
  delay_process_section1_tap0/1 -> out0/1
  in0/1 -> delay_process_section1_tap0/1

== system gm_CustArch_v13/cust_architecture/process_and_retrieve/Filter_ch1/digital_filter/highpass/delay_process_section1_tap1 ==
  in0 : Inport  OutDataTypeStr=fixdt(1, 32, 8)  SampleTime=1
  Enable_out2 : EnablePort  OutDataTypeStr=boolean
  delay_process_section1_tap1 : Delay  DelayLength=double(1)
  out0 : Outport  OutDataTypeStr=fixdt(1, 32, 8)  InitialOutput=0
  wires:
  delay_process_section1_tap1/1 -> out0/1
  in0/1 -> delay_process_section1_tap1/1

== system gm_CustArch_v13/cust_architecture/process_and_retrieve/Filter_ch1/digital_filter/highpass/delay_process_section1_tap11 ==
  in0 : Inport  OutDataTypeStr=fixdt(1, 32, 8)  SampleTime=1
  Enable_out2 : EnablePort  OutDataTypeStr=boolean
  delay_process_section1_tap1 : Delay  DelayLength=double(1)
  out0 : Outport  OutDataTypeStr=fixdt(1, 32, 8)  InitialOutput=0
  wires:
  delay_process_section1_tap1/1 -> out0/1
  in0/1 -> delay_process_section1_tap1/1

== system gm_CustArch_v13/cust_architecture/process_and_retrieve/Filter_ch1/digital_filter/highpass/delay_process_section1_tap12 ==
  in0 : Inport  OutDataTypeStr=fixdt(1, 32, 8)  SampleTime=1
  Enable_out2 : EnablePort  OutDataTypeStr=boolean
  delay_process_section1_tap1 : Delay  DelayLength=double(1)
  out0 : Outport  OutDataTypeStr=fixdt(1, 32, 8)  InitialOutput=0
  wires:
  delay_process_section1_tap1/1 -> out0/1
  in0/1 -> delay_process_section1_tap1/1

== system gm_CustArch_v13/cust_architecture/process_and_retrieve/Filter_ch1/digital_filter/highpass/delay_process_section1_tap13 ==
  in0 : Inport  OutDataTypeStr=fixdt(1, 32, 8)  SampleTime=1
  Enable_out2 : EnablePort  OutDataTypeStr=boolean
  delay_process_section1_tap1 : Delay  DelayLength=double(1)
  out0 : Outport  OutDataTypeStr=fixdt(1, 32, 8)  InitialOutput=0
  wires:
  delay_process_section1_tap1/1 -> out0/1
  in0/1 -> delay_process_section1_tap1/1

== system gm_CustArch_v13/cust_architecture/process_and_retrieve/Filter_ch1/digital_filter/highpass/delay_process_section1_tap14 ==
  in0 : Inport  OutDataTypeStr=fixdt(1, 32, 8)  SampleTime=1
  Enable_out2 : EnablePort  OutDataTypeStr=boolean
  delay_process_section1_tap1 : Delay  DelayLength=double(1)
  out0 : Outport  OutDataTypeStr=fixdt(1, 32, 8)  InitialOutput=0
  wires:
  delay_process_section1_tap1/1 -> out0/1
  in0/1 -> delay_process_section1_tap1/1

== system gm_CustArch_v13/cust_architecture/process_and_retrieve/Filter_ch1/digital_filter/highpass/delay_process_section1_tap15 ==
  in0 : Inport  OutDataTypeStr=fixdt(1, 32, 8)  SampleTime=1
  Enable_out2 : EnablePort  OutDataTypeStr=boolean
  delay_process_section1_tap1 : Delay  DelayLength=double(1)
  out0 : Outport  OutDataTypeStr=fixdt(1, 32, 8)  InitialOutput=0
  wires:
  delay_process_section1_tap1/1 -> out0/1
  in0/1 -> delay_process_section1_tap1/1

== system gm_CustArch_v13/cust_architecture/process_and_retrieve/Filter_ch1/digital_filter/highpass/delay_process_section1_tap16 ==
  in0 : Inport  OutDataTypeStr=fixdt(1, 32, 8)  SampleTime=1
  Enable_out2 : EnablePort  OutDataTypeStr=boolean
  delay_process_section1_tap1 : Delay  DelayLength=double(1)
  out0 : Outport  OutDataTypeStr=fixdt(1, 32, 8)  InitialOutput=0
  wires:
  delay_process_section1_tap1/1 -> out0/1
  in0/1 -> delay_process_section1_tap1/1

== system gm_CustArch_v13/cust_architecture/process_and_retrieve/Filter_ch1/digital_filter/highpass/delay_process_section1_tap17 ==
  in0 : Inport  OutDataTypeStr=fixdt(1, 32, 8)  SampleTime=1
  Enable_out2 : EnablePort  OutDataTypeStr=boolean
  delay_process_section1_tap1 : Delay  DelayLength=double(1)
  out0 : Outport  OutDataTypeStr=fixdt(1, 32, 8)  InitialOutput=0
  wires:
  delay_process_section1_tap1/1 -> out0/1
  in0/1 -> delay_process_section1_tap1/1

== stateflow chart gm_CustArch_v13/cust_architecture/output_interpret/OutputStateMachine/OutputStateMachine ==
  settings: sampleTime=1/1e6  stateMachineType=MOORE_MACHINE  initializeOutput=1
  note: Moore machine
      | State machine to cycle between the different states according
      | to its input variables.
      | The InputState (output of the machine) determines the class of the
      | retrieved data changing its processing in the next steps
  state idle_state
    OutputState=16
  note: The Moore machine output is a function of the current
      | state only. At every time step the input variables dependent
      | on the current state update the output of the state machine.
  state state_magic_number_0
    OutputState=0
  state state_magic_number_01
    OutputState=1
  state state_magic_number_02
    OutputState=2
  state state_magic_number_03
    OutputState=3
  state state_timestamp_0
    OutputState=4
  state state_timestamp_01
    OutputState=5
  state state_DC_sample
    OutputState=6
    count_chs=count_chs+1
  state state_chan_sample
    OutputState=7
  state state_stim_on_off
    OutputState=8
    count_chs=0
    count_stim_on_off=count_stim_on_off+1
  state state_stim_pol
    OutputState=9
    count_stim_on_off=0
    count_stim_pol=count_stim_pol+1
  state state_amp_settle
    OutputState=10
    count_stim_pol=0
    count_amp_settle=count_amp_settle+1
  state state_charge_recov
    OutputState=11
    count_amp_settle=0
    count_state_charge=count_state_charge+1
  state state_DAC
    OutputState=12
    count_state_charge=0
    count_1=count_1+1
  state state_ADC
    OutputState=13
    count_1=0
    count_2=count_2+1
  state state_TTL_in
    count_2=0
    OutputState=14
  state state_TTL_out
    OutputState=15
  (default) -> idle_state
  state_TTL_out -> idle_state
  idle_state -> state_magic_number_0 : [input_state==8]
  state_magic_number_0 -> state_magic_number_01
  state_magic_number_01 -> state_magic_number_02
  state_magic_number_02 -> state_magic_number_03
  state_magic_number_03 -> state_timestamp_0
  state_timestamp_0 -> state_timestamp_01
  state_timestamp_01 -> state_DC_sample
  state_chan_sample -> state_DC_sample [order 1] : [count_chs<160]
  state_DC_sample -> state_chan_sample
  state_chan_sample -> state_stim_on_off [order 2] : [count_chs==160]
  state_stim_on_off -> state_stim_pol : [count_stim_on_off==8]
  state_stim_pol -> state_amp_settle : [count_stim_pol==8]
  state_amp_settle -> state_charge_recov : [count_amp_settle==8]
  state_charge_recov -> state_DAC : [count_state_charge==8]
  state_DAC -> state_DAC [order 2]
  state_DAC -> state_ADC [order 1] : [count_1==8]
  state_ADC -> state_ADC [order 2]
  state_ADC -> state_TTL_in [order 1] : [count_2==8]
  state_TTL_in -> state_TTL_out
  data: OutputState output uint8 =uint8(0); count_1 local uint8 =uint8(0); count_2 local uint8 =uint8(0); input_state input uint8; count_stim_pol local uint8 =uint8(0); count_stim_on_off local uint8 =uint8(0); count_amp_settle local uint8 =uint8(0); count_state_charge local uint8 =uint8(0); count_chs local uint8 =uint8(0)
